simulink model "calefaccion_control_prueba_r2020a"  (R2020a)
settings: Solver=VariableStepAuto  StartTime=0.0  StopTime=30  MaxStep=20*(1/60)*(1/24)  RelTol=1e-3
values from neighbouring files (symbols this model uses):
  Tref = 16.5    [izaro_script.m]
libraries: simulink x1
settings Model: Creator=izaro.garro  LastModifiedBy=djoroya
settings SFSimCC: CustomCodeUndefinedFunction=UseInterfaceOnly

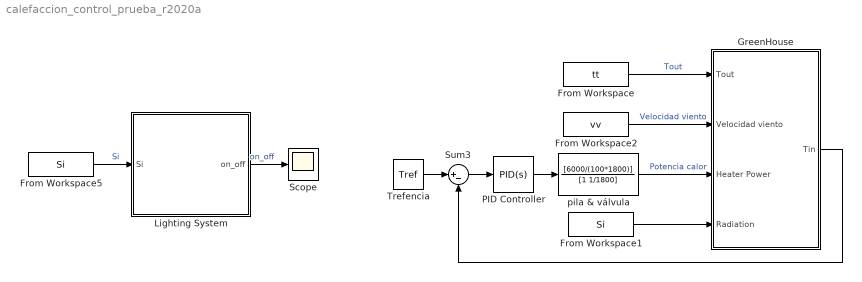
== system calefaccion_control_prueba_r2020a ==
  From Workspace : FromWorkspace  VariableName=tt  ZeroCross=off
  From Workspace1 : FromWorkspace  VariableName=Si  ZeroCross=off
  From Workspace2 : FromWorkspace  VariableName=vv  ZeroCross=off
  From Workspace5 : FromWorkspace  VariableName=Si  ZeroCross=off
  GreenHouse : Subsystem
  "Lighting System " : Subsystem  mask{MinRadAcum=5e6, MaxDuration=5, RadMaxPower=4*200}
      mask prompts: MinRadAcum "Minimum Acumulated Radiation (J)"; MaxDuration "Maximum Duration (hours)"; RadMaxPower "Radiation Power (W)"
  PID Controller : simulink/Continuous/PID Controller  Controller=PID  Form=Parallel  TimeDomain=Continuous-time  UseExternalTs=off  SampleTime=-1  IntegratorMethod=Forward Euler  FilterMethod=Forward Euler  ControllerParametersSource=internal  P=2  I=2/1200  D=0  UseFilter=on  N=0.0006  TunerSelectOption=Transfer Function Based (PID Tuner App)  ZeroCross=off  InitialConditionSource=internal  InitialConditionForIntegrator=0  InitialConditionForFilter=0  DifferentiatorICPrevScaledInput=0  ExternalReset=none  TrackingMode=off  Kt=1  LimitOutput=on  UpperSaturationLimit=100  LowerSaturationLimit=0  LinearizeAsGain=on  AntiWindupMode=clamping  Kb=1  POutMin=[]  POutMax=[]  IOutMin=[]  IOutMax=[]  DOutMin=[]  DOutMax=[]  NOutMin=[]  NOutMax=[]  SumOutMin=[]  SumOutMax=[]  SaturationOutMin=[]  SaturationOutMax=[]  PParamMin=[]  PParamMax=[]  IParamMin=[]  IParamMax=[]  DParamMin=[]  DParamMax=[]  NParamMin=[]  NParamMax=[]  KbParamMin=[]  KbParamMax=[]  KtParamMin=[]  KtParamMax=[]  KbOutMin=[]  KbOutMax=[]  KtOutMin=[]  KtOutMax=[]  IntegratorOutMin=[]  IntegratorOutMax=[]  FilterOutMin=[]  FilterOutMax=[]  SumI1OutMin=[]  SumI1OutMax=[]  SumI2OutMin=[]  SumI2OutMax=[]  SumI3OutMin=[]  SumI3OutMax=[]  SumI4OutMin=[]  SumI4OutMax=[]  SumDOutMin=[]  SumDOutMax=[]  DifferentiatorOutMin=[]  DifferentiatorOutMax=[]  FilterDiffOutCoefMin=[]  FilterDiffOutCoefMax=[]  ReciprocalOutMin=[]  ReciprocalOutMax=[]  SumDenOutMin=[]  SumDenOutMax=[]  SumNumOutMin=[]  SumNumOutMax=[]  DivideOutMin=[]  DivideOutMax=[]  UdiffTsProdOutMin=[]  UdiffTsProdOutMax=[]  NTsProdOutMin=[]  NTsProdOutMax=[]  UintegralTsProdOutMin=[]  UintegralTsProdOutMax=[]  UngainTsProdOutMin=[]  UngainTsProdOutMax=[]  IntegratorContinuousStateAttributes=''  IntegratorStateMustResolveToSignalObject=off  IntegratorRTWStateStorageClass=Auto  FilterContinuousStateAttributes=''  FilterStateMustResolveToSignalObject=off  FilterRTWStateStorageClass=Auto  ParallelPVariant=InternalParameters  IdealPVariant=Disabled  IVariant=InternalParameters  DVariant=InternalParameters  IntegratorVariant=Continuous  SatVariant=Enabled  AWVariant=ContClampingParallel  PCopyVariant=Disabled  TRVariant=Disabled  FdbkBlocksVariant=Forward  IdealPFdbkVariant=Disabled  SatFdbkVariant=Disabled  DerivativeFilterVariant=ContFilter  NVariant=InternalParameters  NCopyVariant=Disabled  FilterICVariant=InternalICsFilter  IntegratorICVariant=InternalICs  ExternalResetVariant=Disabled  TRSumVariant=Passthrough  SumFdbkVariant=Disabled  SumVariant=Sum_PID  TsampFilterVariant=InternalTs  TsampNgainVariant=Passthrough  TsampIntegralVariant=Passthrough
  Scope : Scope
  Sum3 : Sum  Inputs=|+-
  Trefencia : Constant  Value=Tref
  pila & válvula : TransferFcn  Numerator=[6000/(100*1800)]  Denominator=[1 1/1800]
  wires:
  Sum3/1 -> PID Controller/1
  PID Controller/1 -> pila & válvula/1
  Trefencia/1 -> Sum3/1
  From Workspace/1 -> GreenHouse/1(Tout)  "Tout"
  From Workspace2/1 -> GreenHouse/2(Velocidad viento)  "Velocidad viento"
  pila & válvula/1 -> GreenHouse/3(Heater Power)  "Potencia calor"
  From Workspace1/1 -> GreenHouse/4(Radiation)
  GreenHouse/1(Tin) -> Sum3/2
  From Workspace5/1 -> "Lighting System "/1(Si)  "Si"
  "Lighting System "/1(on_off) -> Scope/1  "on_off"

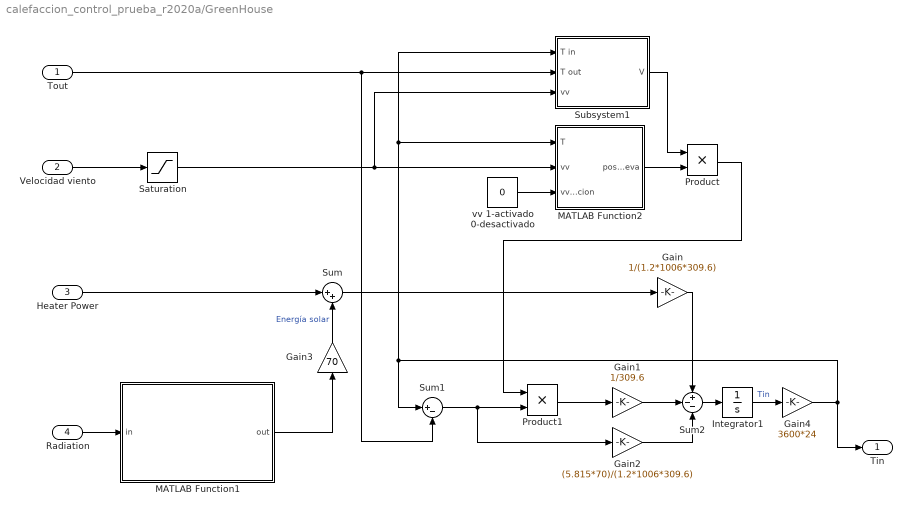
== system calefaccion_control_prueba_r2020a/GreenHouse ==
  Tout : Inport
  Velocidad viento : Inport  Port=2
  Heater Power : Inport  Port=3
  Radiation : Inport  Port=4
  Gain : Gain  Gain=1/(1.2*1006*309.6)
  Gain1 : Gain  Gain=1/309.6
  Gain2 : Gain  Gain=(5.815*70)/(1.2*1006*309.6)
  Gain3 : Gain  Gain=70
  Gain4 : Gain  Gain=3600*24
  Integrator1 : Integrator  InitialCondition=20
  MATLAB Function1 : MATLAB Function  TreatAsAtomicUnit=on  SystemSampleTime=600
  MATLAB Function2 : MATLAB Function  TreatAsAtomicUnit=on  SystemSampleTime=1
  Product : Product
  Product1 : Product
  Saturation : Saturate  UpperLimit=Inf  LowerLimit=0
  Subsystem1 : Subsystem
      mask Display: image('$imagefile'); % Use "Edit Image" on toolstrip to change.
  Sum : Sum  Inputs=|++
  Sum1 : Sum  Inputs=|+-
  Sum2 : Sum  Inputs=+--
  vv 1-activado 0-desactivado : Constant  Value=0
  Tin : Outport
  wires:
  Gain1/1 -> Sum2/2
  Gain3/1 -> Sum/2  "Energía solar"
  Sum1/1 -> Gain2/1, Product1/2
  Subsystem1/1(V) -> Product/1
  Gain/1 -> Sum2/1
  Gain2/1 -> Sum2/3
  Product/1 -> Product1/1
  Sum/1 -> Gain/1
  Sum2/1 -> Integrator1/1
  MATLAB Function2/1(posicionNueva) -> Product/2
  Radiation/1 -> MATLAB Function1/1(in)
  MATLAB Function1/1(out) -> Gain3/1
  vv 1-activado 0-desactivado/1 -> MATLAB Function2/3(vv_opcion)
  Tout/1 -> Subsystem1/2(T out), Sum1/2
  Integrator1/1 -> Gain4/1  "Tin"
  Product1/1 -> Gain1/1
  Heater Power/1 -> Sum/1
  Velocidad viento/1 -> Saturation/1
  Gain4/1 -> Subsystem1/1(T in), MATLAB Function2/1(T), Sum1/1, Tin/1
  Saturation/1 -> Subsystem1/3(vv), MATLAB Function2/2(vv)

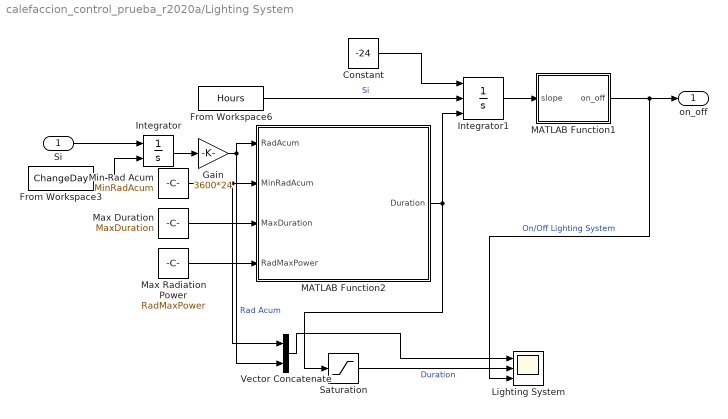
== system calefaccion_control_prueba_r2020a/Lighting System  ==
  Si : Inport
  Constant : Constant  Value=-24
  From Workspace3 : FromWorkspace  VariableName=ChangeDay
  From Workspace6 : FromWorkspace  VariableName=Hours  ZeroCross=off
  Gain : Gain  Gain=3600*24
  Integrator : Integrator  ExternalReset=rising
  Integrator1 : Integrator  ExternalReset=rising  InitialConditionSource=external
  Lighting System : Scope  NumInputPorts=3
  MATLAB Function1 : MATLAB Function  TreatAsAtomicUnit=on
  MATLAB Function2 : MATLAB Function  TreatAsAtomicUnit=on
  Max Duration : Constant  Value=MaxDuration
  Max Radiation Power : Constant  Value=RadMaxPower
  Min Rad Acum : Constant  Value=MinRadAcum
  Saturation : Saturate  UpperLimit=Inf  LowerLimit=0
  Vector Concatenate : Concatenate
  on_off : Outport
  wires:
  MATLAB Function1/1(on_off) -> Lighting System/3, on_off/1  "On/Off Lighting System"
  Integrator/1 -> Gain/1
  MATLAB Function2/1(Duration) -> Saturation/1, Integrator1/3
  Si/1 -> Integrator/1
  Max Duration/1 -> MATLAB Function2/3(MaxDuration)
  Integrator1/1 -> MATLAB Function1/1(slope)
  Min Rad Acum/1 -> Vector Concatenate/1, MATLAB Function2/2(MinRadAcum)
  From Workspace6/1 -> Integrator1/2  "Si"
  From Workspace3/1 -> Integrator/2
  Constant/1 -> Integrator1/1
  Gain/1 -> Vector Concatenate/2, MATLAB Function2/1(RadAcum)  "Rad Acum"
  Vector Concatenate/1 -> Lighting System/1
  Saturation/1 -> Lighting System/2  "Duration"
  Max Radiation Power/1 -> MATLAB Function2/4(RadMaxPower)

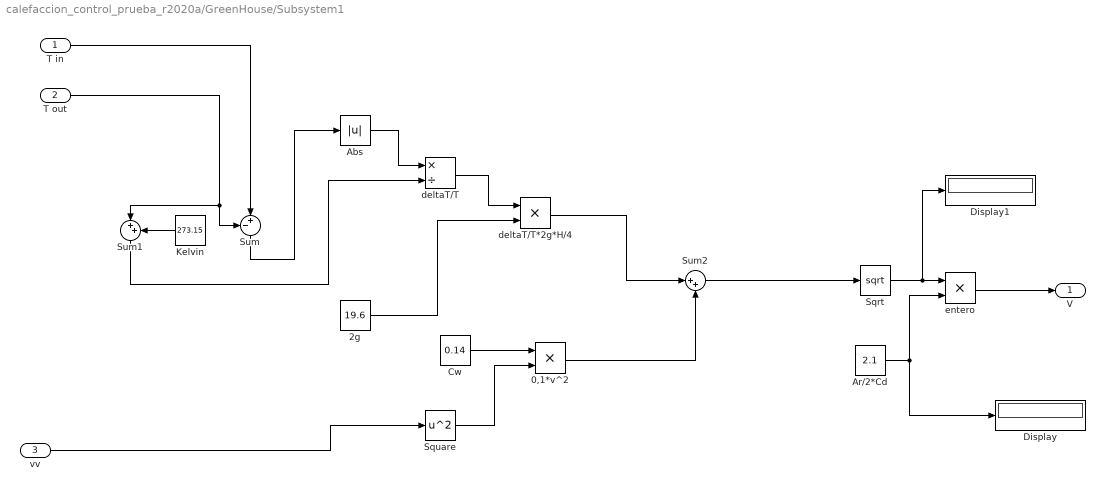
== system calefaccion_control_prueba_r2020a/GreenHouse/Subsystem1 ==
  T in : Inport
  T out : Inport  Port=2
  vv : Inport  Port=3
  0,1*v^2 : Product  Inputs=**
  2g : Constant  Value=19.6
  Abs : Abs
  Ar/2*Cd : Constant  Value=2.1
  Cw : Constant  Value=0.14
  Display : Display
  Display1 : Display
  Kelvin : Constant  Value=273.15
  Sqrt : Sqrt  SaturateOnIntegerOverflow=on
  Square : Math  Operator=square  SignedPower=on  SaturateOnIntegerOverflow=on
  Sum : Sum  Inputs=-+|
  Sum1 : Sum  Inputs=|++
  Sum2 : Sum  Inputs=|++
  deltaT/T : Product  Inputs=*/
  deltaT/T*2g*H/4 : Product  Inputs=**
  entero : Product  Inputs=**
  V : Outport
  wires:
  T in/1 -> Sum/2
  Sum2/1 -> Sqrt/1
  Square/1 -> 0,1*v^2/2
  Cw/1 -> 0,1*v^2/1
  deltaT/T/1 -> deltaT/T*2g*H/4/1
  Sum1/1 -> deltaT/T/2
  Kelvin/1 -> Sum1/2
  T out/1 -> Sum1/1, Sum/1
  Ar/2*Cd/1 -> Display/1, entero/2
  deltaT/T*2g*H/4/1 -> Sum2/1
  2g/1 -> deltaT/T*2g*H/4/2
  0,1*v^2/1 -> Sum2/2
  Sqrt/1 -> Display1/1, entero/1
  entero/1 -> V/1
  vv/1 -> Square/1
  Abs/1 -> deltaT/T/1
  Sum/1 -> Abs/1

== matlab function calefaccion_control_prueba_r2020a/GreenHouse/MATLAB Function1 ==
  settings: updateMethod=DISCRETE
  data: in input; out output
function out = pantallasombreo(in)

persistent flag;

if isempty(flag)
    flag = 0;
end

if in<15
    out=0;
    flag=0;
    
elseif in<=250
    out=in*0.95;
    flag=0;
elseif in>=300
    out=in*0.5;
    flag=1;
else
    if flag==1
        out=in*0.5;
    else
        out=in*0.95;
    end
end

== matlab function calefaccion_control_prueba_r2020a/GreenHouse/MATLAB Function2 ==
  settings: updateMethod=DISCRETE
  data: T input; posicionNueva output; vv input; vv_opcion input
function posicionNueva  = ventanas(T,vv,vv_opcion)

persistent posicionAnterior;

if isempty(posicionAnterior)
    posicionAnterior = 0;
end


posicionIdeal = CalcularPosicion(T, 20);

if abs(posicionIdeal - posicionAnterior) < 0.1
    posicionNueva = posicionAnterior;   
else
    if posicionIdeal > posicionAnterior
        posicionNueva = posicionAnterior + 0.1;
    else
        posicionNueva = posicionAnterior - 0.1;
    end
end

if vv_opcion==1
    if vv>10 && posicionNueva>0.3
        posicionNueva=0.3;
    end
end

posicionAnterior = posicionNueva;
end

function apertura= CalcularPosicion(temperatura, consigna)
if temperatura > consigna
    apertura = (temperatura - consigna) / 10;
    if apertura > 1
        apertura = 1;
    end
else
    apertura = 0;
end
end

== matlab function calefaccion_control_prueba_r2020a/Lighting System /MATLAB Function2 ==
  data: RadAcum input; Duration output; MinRadAcum input; MaxDuration input; RadMaxPower input
function Duration = fcn(RadAcum,MinRadAcum,MaxDuration,RadMaxPower)



Duration = (1/RadMaxPower)*(MinRadAcum-RadAcum);
Duration = Duration/3600;
Duration = min(MaxDuration,Duration);

== matlab function calefaccion_control_prueba_r2020a/Lighting System /MATLAB Function1 ==
  data: slope input; on_off output
function on_off = fcn(slope)

on_off = 0.5+0.5*sign(slope);
